simulink model "cruise_control_statemachine"  (R2018a)
settings: Solver=FixedStepAuto  StartTime=0.0  StopTime=inf  RelTol=1e-3  EnableMultiTasking=on
undefined symbols (not defined in the file): Angular, Linear
libraries: robotlib x2
settings Model: Creator=ece446  LastModifiedBy=Ivory - rahulbhadani
settings OptimizationCC: LifeSpan=Inf  MaxStackSize=64
settings DebuggingCC: SFUnexpectedBacktrackingDiag=warning  SFNoUnconditionalDefaultTransitionDiag=warning  SFExecutionAtInitializationDiag=none
settings HardwareCC: ProdBitPerPointer=32  ProdBitPerSizeT=32  ProdBitPerPtrDiffT=32  ProdLargestAtomicFloat=None  ProdIntDivRoundTo=Undefined  ProdEndianess=Unspecified  ProdWordSize=32  ProdHWDeviceType=Generic->Unspecified (assume 32-bit Generic)  UseEmbeddedCoderFeatures=off
settings RTWCC: SystemTargetFile=ert.tlc  HardwareBoard=Robot Operating System (ROS)  TLCOptions=-aInlineSetEventsForThisBaseRateFcn=TLC_FALSE -aSuppressMultiTaskScheduler=TLC_FALSE -aRateBasedStepFcn=0  TemplateMakefile=ert_default_tmf  GenerateReport=on  Toolchain=Catkin  LaunchReport=on  TargetLang=C++
settings CodeAppCC: ForceParamTrailComments=on  OperatorAnnotations=on  StateflowObjectComments=on  MATLABSourceComments=on
settings ERTTargetCC: MultiwordLength=2048  ERTCustomFileBanners=off  SupportContinuousTime=on  SupportNonInlinedSFcns=on  RemoveResetFunc=off  ModelStepFunctionPrototypeControlCompliant=off
settings ConfigComp: CovMetricSettings=dw  CovHtmlReporting=on  CovSaveCumulativeToWorkspaceVar=on  CovSaveSingleToWorkspaceVar=on  CovExternalEMLEnable=off

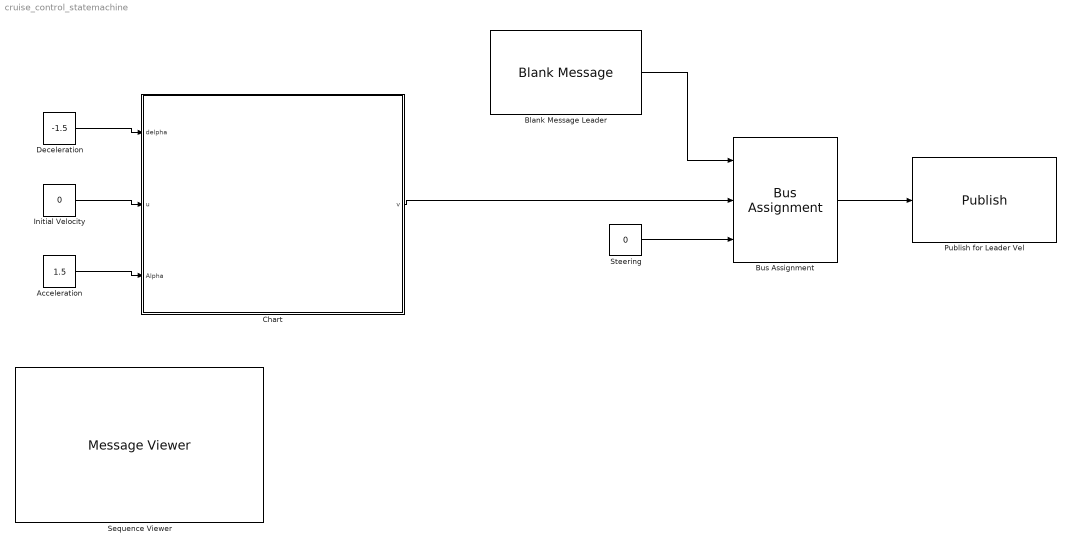
== system cruise_control_statemachine ==
  Acceleration : Constant  Value=1.5
  Blank Message Leader : robotlib/Blank Message  SourceLibraryInfo=This block requires Robotics System Toolbox  messageType=geometry_msgs/Twist  SampleTime=inf
      settings: SourceProductBaseCode=RO
  Bus Assignment : BusAssignment  AssignedSignals=Linear.X,Angular.Z
  Chart : Stateflow chart  TreatAsAtomicUnit=on
  Deceleration : Constant  Value=-1.5
  Initial Velocity : Constant  Value=0
  Publish for Leader Vel : robotlib/Publish  SourceLibraryInfo=This block requires Robotics System Toolbox  topicSource=Specify your own  topic=cmd_vel  messageType=geometry_msgs/Twist  messageQueueLength=1
      settings: SourceProductBaseCode=RO
  Sequence Viewer : MessageViewer
  Steering : Constant  Value=0
  wires:
  Blank Message Leader/1 -> Bus Assignment/1
  Bus Assignment/1 -> Publish for Leader Vel/1
  Steering/1 -> Bus Assignment/3
  Chart/1(v) -> Bus Assignment/2
  Deceleration/1 -> Chart/1(delpha)
  Acceleration/1 -> Chart/3(Alpha)
  Initial Velocity/1 -> Chart/2(u)

== stateflow chart cruise_control_statemachine/Chart ==
  state DecelerateTo35
    entry: entryState = nextState; v = u2;
    during: v = getNewV(v, delpha);
    exit: nextState = entryState + 1;
    note: STATE 2
  state AccelerateTo55_init
    entry: entryState = 1; v = u;
    during: v = getNewV(v, Alpha)
    exit:  nextState = entryState + 1;
    note: STATE 1
  state Hold
    entry: u2 = v;
    during: v = u2;
    exit:
    note: HOLD STATE
  state AccelerateTo55
    entry: entryState = nextState; v = u2;
    during: v = getNewV(v, Alpha);
    exit: nextState = entryState + 1;
    note: STATE 3, 5
  state zero
    entry: v = 0;
    during:v = 0;
    note: STATE 12
  state DecelerateTo0
    entry: entryState = nextState; v= u2;
    during: v = getNewV(v, delpha);
    exit: nextState = entryState + 1;
    note: STATE 11
  state DecelerateTo45
    entry: entryState = nextState; v = u2;
    during: v = getNewV(v, delpha);
    exit: nextState = entryState + 1;
    note: STATE 4
  DecelerateTo35 -> Hold : [v <= 35]
  Hold -> DecelerateTo35 [order 1] : [after(60, sec) && entryState == 1]
  (default) -> AccelerateTo55_init
  AccelerateTo55_init -> Hold : [v>=55 ]
  Hold -> AccelerateTo55 [order 2] : [after(60, sec) && (entryState == 2 || entryState == 4)]
  Hold -> DecelerateTo0 [order 4] : [after(60, sec) && entryState== 5]
  AccelerateTo55 -> Hold : [v >= 55]
  DecelerateTo0 -> zero : [v <=0]
  DecelerateTo45 -> Hold : [v <= 45]
  Hold -> DecelerateTo45 [order 3] : [after(60, sec) && entryState == 3]
  data: init_velocity function_input; acceleration function_input; new_vel function_output; delpha input; u input; Alpha input; v output =0; u2 local =0; entryState local =0; nextState local =0
  function new_vel = getNewV(init_velocity, acceleration):
    | function new_vel = getNewV(init_velocity, acceleration)
    | 
    | new_vel = init_velocity + (acceleration*0.05);
    | 
    | end
